simulink model "Storage_Cell"  (R2021b)
settings: Solver=VariableStepAuto  StartTime=0.0  StopTime=1  RelTol=1e-3
values from neighbouring files (symbols this model uses):
  dUdc = 0.1    [Storage_Cell_m.m]
  FFT_N = FFT_T / FFT_T_sample    (= 50)    [Storage_Cell_m.m]
  FFT_T_sample = 1/FFT_F_sample    (= 0.0002)    [Storage_Cell_m.m]
  Timesample = 1/(4*Fpwm)    (= 5e-05)    [Storage_Cell_m.m]
  Tpwm = 1/Fpwm    (= 0.0002)    [Storage_Cell_m.m]
  Udc = 450    [Storage_Cell_m.m]
  Us = 320    [Storage_Cell_m.m]
  Us_max = 380    [Storage_Cell_m.m]
libraries: spsSeriesRLCBranchLib x19, spsIGBTDiodeLib x10, spsVoltageMeasurementLib x10, spsSawtoothGeneratorLib x7, spsCurrentMeasurementLib x5, spsDCVoltageSourceLib x5, spspowerguiLib x1
settings Model: Creator=user  LastModifiedBy=mrsas

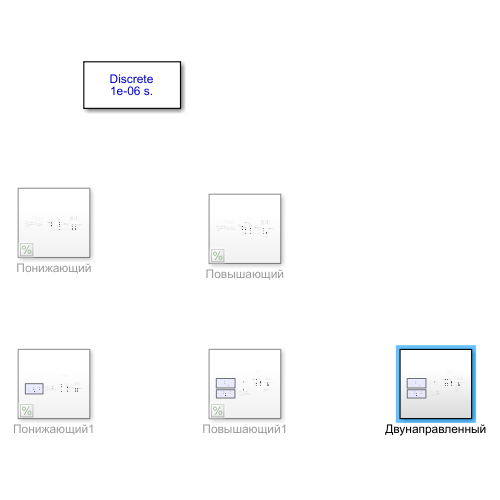
[thumbnail: Simulink's stored preview of the top-level diagram]
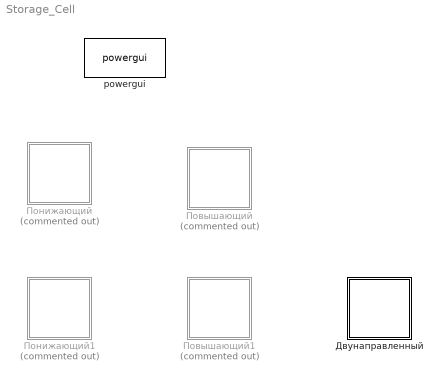
== system Storage_Cell ==
  powergui : spspowerguiLib/powergui  Priority=1  SimulationMode=Discrete  SampleTime=1e-6  frequency=60  Iterations=50  frequencyindice=0  Pbase=100e6  ErrMax=1e-4  UnitsV=kV  UnitsW=MW  buscounter=0  FunctionMessages=off  echomessages=off  EnableUseOfTLC=off  CurrentSourceSwitches=off  DisableSnubberDevices=off  DisableRonSwitches=off  DisableVfSwitches=off  DisplayEquations=off  AutomaticDiscreteSolvers=off  SolverType=Tustin/Backward Euler (TBE)  Interpol=off  ExternalGateDelay=off  methode=off  Ts=100  x0status=blocks  SPID=on  SwTol=0  HookPort=off  NonlinearTolerance=1e-4  nMaxIteration=100  ContinueOnMaxIteration=off  RestoreLinks=warning  ResistiveCurrentMeasurement=off  Frange=[0:2:500]  Ylog=off  Xlog=on  ShowGrid=off  save=off  variable=ZData  structure=0  ZoomFFT=off  StartTime=0.0  cycles=1  DisplayStyle=1  fundamental=60  FreqAxis=off  MaxFrequency=1000  frequencyindicesteady=1  RmsSteady=1  display=off
  Двунаправленный : Subsystem
  Повышающий : Subsystem  Commented=on
  Повышающий1 : Subsystem  Commented=on
  Понижающий : Subsystem  Commented=on
  Понижающий1 : Subsystem  Commented=on

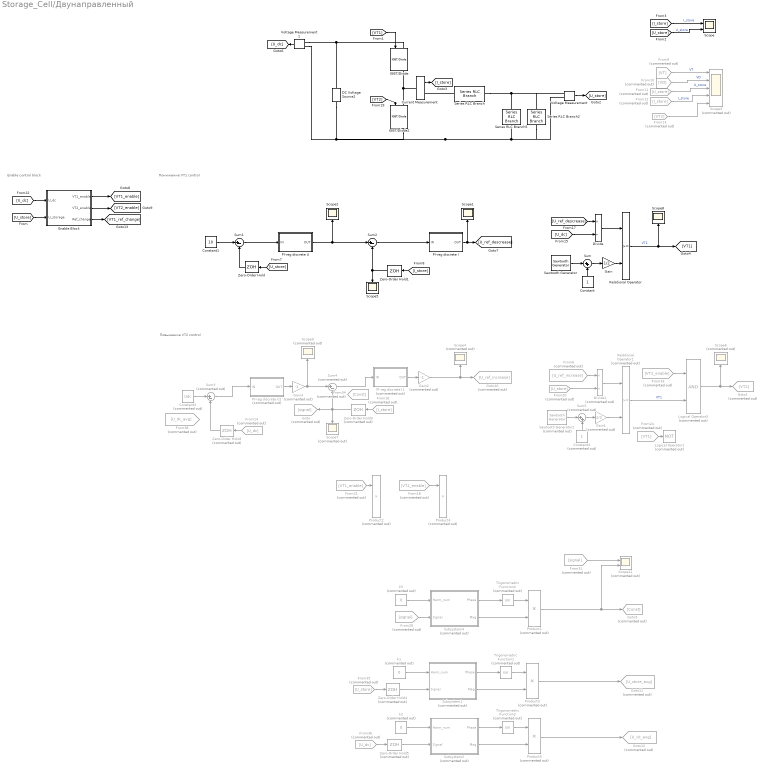
== system Storage_Cell/Двунаправленный ==
  note: Enable control block
  note: Повышение
      | VT2 control
  note: Понижение
      | VT1 control
  Constant : Constant
  Constant1 : Constant  Value=10
  Constant3 : Constant  Commented=on  Value=Udc
  Constant4 : Constant  Commented=on
  Current Measurement : spsCurrentMeasurementLib/Current Measurement  PhasorSimulation=off  OutputType=Complex  PSBequivalent=0
  DC Voltage Source2 : spsDCVoltageSourceLib/DC Voltage Source  Amplitude=20  Measurements=None
  Divide : Product  Inputs=*/
  Divide1 : Product  Commented=on  Inputs=*/
  Enable Block : Subsystem
  From10 : From  Commented=on  GotoTag=VD
  From11 : From  Commented=on  GotoTag=U_store
  From12 : From  Commented=on  GotoTag=I_store
  From13 : From  Commented=on  GotoTag=VT2
  From14 : From  Commented=on  GotoTag=U_dc
  From16 : From  Commented=on  GotoTag=I_store
  From18 : From  Commented=on  GotoTag=VT2_enable
  From20 : From  Commented=on  GotoTag=U_store
  From21 : From  Commented=on  GotoTag=VT1_enable
  From24 : From  Commented=on  GotoTag=VT1
  From28 : From  Commented=on  GotoTag=signal
  From31 : From  Commented=on  GotoTag=signal
  From33 : From  Commented=on  GotoTag=VT2_enable
  From34 : From  Commented=on  GotoTag=Const
  From35 : From  Commented=on  GotoTag=U_store
  From36 : From  Commented=on  GotoTag=U_dc
  From38 : From  Commented=on  GotoTag=U_dc_avg
  From6 : From  Commented=on  GotoTag=U_ref_increase
  From9 : From  Commented=on  GotoTag=VT
  Gain : Gain  Gain=1/2
  Gain1 : Gain  Commented=on  Gain=1/2
  Gain2 : Gain  Commented=on  Gain=-1
  Gain4 : Gain  Commented=on  Gain=-1
  Goto : Goto  Commented=on  GotoTag=signal
  Goto1 : Goto  Commented=on  GotoTag=VT2
  Goto10 : Goto  Commented=on  GotoTag=U_ref_increase
  Goto11 : Goto  Commented=on  GotoTag=U_store_avg
  Goto12 : Goto  Commented=on  GotoTag=U_dc_avg
  Goto5 : Goto  Commented=on  GotoTag=Const
  IGBT/Diode : spsIGBTDiodeLib/IGBT//Diode  Ron=1e-3  Rs=1e5  Cs=inf  Measurements=on
  IGBT/Diode2 : spsIGBTDiodeLib/IGBT//Diode  Ron=1e-3  Rs=1e5  Cs=inf  Measurements=on
  Logical Operator1 : Logic  Commented=on  Operator=NOT  AllPortsSameDT=off  OutDataTypeStr=boolean
  Logical Operator5 : Logic  Commented=on  AllPortsSameDT=off  OutDataTypeStr=boolean
  PI-reg discrete I : Subsystem  mask{First_condition=0, T=0.003, K=7.5, min=0, max=20, dt=Tpwm}
      mask prompts: T "Integral"; K "Proportional"; min "saturation_min"; max "saturation_max"; dt "timesample"
  PI-reg discrete I1 : Subsystem  Commented=on  mask{First_condition=370, T=0.001/0.1, K=3, min=-400, max=400, dt=Timesample}
      mask prompts: T "Integral"; K "Proportional"; min "saturation_min"; max "saturation_max"; dt "timesample"
  PI-reg discrete U : Subsystem  mask{First_condition=0, T=0.01, K=0.5, min=0, max=4, dt=Tpwm}
      mask prompts: T "Integral"; K "Proportional"; min "saturation_min"; max "saturation_max"; dt "timesample"
  PI-reg discrete U1 : Subsystem  Commented=on  mask{First_condition=0, T=0.1, K=0.1, min=-1000, max=1000, dt=Timesample}
      mask prompts: T "Integral"; K "Proportional"; min "saturation_min"; max "saturation_max"; dt "timesample"
  Product{1..5} (5 alike) : Product  Commented=on
  Relational Operator : RelationalOperator  OutDataTypeStr=boolean  RndMeth=Simplest
  Relational Operator1 : RelationalOperator  Commented=on  OutDataTypeStr=boolean  RndMeth=Simplest
  Sawtooth Generator : spsSawtoothGeneratorLib/Sawtooth Generator  Freq=Fpwm  Phase=0  Ts=0
  Sawtooth Generator1 : spsSawtoothGeneratorLib/Sawtooth Generator  Commented=on  Freq=Fpwm  Phase=0  Ts=0
  Scope : Scope  NumInputPorts=2
  Scope{1..2,5,8} (4 alike) : Scope
  Scope11 : Scope  Commented=on  NumInputPorts=2
  Scope3 : Scope  Commented=on  NumInputPorts=5
  Scope{4,6..7,9} (4 alike) : Scope  Commented=on
  Series RLC Branch : spsSeriesRLCBranchLib/Series RLC Branch  LConnTagsString=__new0  RConnTagsString=__new0  BranchType=RL  Resistance=0.1  Inductance=3e-3  SetiL0=on  InitialCurrent=0  Capacitance=1e-6  Setx0=off  InitialVoltage=0  Measurements=None
  Series RLC Branch2 : spsSeriesRLCBranchLib/Series RLC Branch  LConnTagsString=__new0  RConnTagsString=__new0  BranchType=R  Resistance=5  Inductance=1e-3  SetiL0=off  InitialCurrent=0  Capacitance=1000e-6  Setx0=on  InitialVoltage=0  Measurements=None
  Series RLC Branch5 : spsSeriesRLCBranchLib/Series RLC Branch  LConnTagsString=__new0  RConnTagsString=__new0  BranchType=C  Resistance=1  Inductance=1e-3  SetiL0=off  InitialCurrent=0  Capacitance=680e-6  Setx0=on  InitialVoltage=0  Measurements=None
  Subsystem1 : Subsystem  Commented=on
  Subsystem2 : Subsystem  Commented=on
  Subsystem4 : Subsystem  Commented=on
  Sum : Sum  Inputs=|++
  Sum1 : Sum  Inputs=|+-
  Sum2 : Sum  Inputs=|+-
  Sum3 : Sum  Commented=on  Inputs=|+-
  Sum4 : Sum  Commented=on  Inputs=|+-
  Sum5 : Sum  Commented=on  Inputs=|++
  Trigonometric Function1 : Trigonometry  Commented=on
  Trigonometric Function2 : Trigonometry  Commented=on
  Trigonometric Function4 : Trigonometry  Commented=on
  Voltage Measurement : spsVoltageMeasurementLib/Voltage Measurement  PhasorSimulation=off  OutputType=Complex  PSBequivalent=0
  Voltage Measurement1 : spsVoltageMeasurementLib/Voltage Measurement  PhasorSimulation=off  OutputType=Complex  PSBequivalent=0
  Zero-Order Hold : ZeroOrderHold  SampleTime=Timesample
  Zero-Order Hold1 : ZeroOrderHold  SampleTime=Timesample
  Zero-Order Hold{2..5} (4 alike) : ZeroOrderHold  Commented=on  SampleTime=Timesample
  k1 : Constant  Commented=on  Value=0
  k2 : Constant  Commented=on  Value=0
  k5 : Constant  Commented=on  Value=0
  wires:
  Gain2/1 -> Goto10/1, Scope4/1
  Gain4/1 -> Scope9/1, Sum4/1
  Divide1/1 -> Relational Operator1/1
  Sum3/1 -> PI-reg discrete U1/1(IN)
  Zero-Order Hold3/1 -> Sum4/2, Goto/1, Scope7/1
  PI-reg discrete U1/1(OUT) -> Gain4/1
  PI-reg discrete I1/1(OUT) -> Gain2/1
  Divide/1 -> Relational Operator/1
  Sum/1 -> Gain/1
  Current Measurement/1 -> [I_store]
  Gain/1 -> Relational Operator/2
  Sawtooth Generator/1 -> Sum/1
  Voltage Measurement1/1 -> [U_dc]
  Voltage Measurement/1 -> [U_store]
  Constant/1 -> Sum/2
  [U_ref_descrease] -> Divide/1
  Relational Operator/1 -> Scope8/1, [VT1]  "VT1"
  [VT1] -> IGBT/Diode/1
  PI-reg discrete I/1(OUT) -> [U_ref_descrease], Scope1/1
  [U_store] -> Zero-Order Hold/1
  Zero-Order Hold1/1 -> Scope5/1, Sum2/2
  [I_store] -> Zero-Order Hold1/1
  From9/1 -> Scope3/1  "VT"
  From10/1 -> Scope3/2  "VD"
  From11/1 -> Scope3/3  "U_store"
  From12/1 -> Scope3/4  "I_store"
  From13/1 -> Scope3/5
  Constant3/1 -> Sum3/1
  From14/1 -> Zero-Order Hold2/1
  Zero-Order Hold2/1 -> Sum3/2
  [U_dc] -> Divide/2
  From16/1 -> Zero-Order Hold3/1
  From20/1 -> Divide1/2
  From6/1 -> Divide1/1
  Constant4/1 -> Sum5/2
  Sawtooth Generator1/1 -> Sum5/1
  Gain1/1 -> Relational Operator1/2
  Sum5/1 -> Gain1/1
  [VT2] -> IGBT/Diode2/1
  [U_dc] -> Enable Block/1(U_dc)
  [U_store] -> Enable Block/2(U_storage)
  Enable Block/1(VT1_enable) -> [VT1_enable]
  Enable Block/2(VT2_enable) -> [VT2_enable]
  Enable Block/3(Ref_change) -> [VT1_ref_change]
  Sum1/1 -> PI-reg discrete U/1(IN)
  Constant1/1 -> Sum1/1
  Sum2/1 -> PI-reg discrete I/1(IN)
  Sum4/1 -> PI-reg discrete I1/1(IN)
  Relational Operator1/1 -> Logical Operator5/2  "VT1"
  From33/1 -> Logical Operator5/1
  Logical Operator5/1 -> Goto1/1, Scope6/1
  From18/1 -> Product4/1
  From21/1 -> Product2/1
  From24/1 -> Logical Operator1/1
  k5/1 -> Subsystem4/1(Harm_num)
  From28/1 -> Subsystem4/2(Signal)
  Product1/1 -> Scope11/2, Goto5/1
  Subsystem4/2(Mag) -> Product1/2
  Subsystem4/1(Phase) -> Trigonometric Function4/1
  Trigonometric Function4/1 -> Product1/1
  From31/1 -> Scope11/1
  From35/1 -> Zero-Order Hold4/1
  Trigonometric Function1/1 -> Product3/1
  Subsystem1/1(Phase) -> Trigonometric Function1/1
  Subsystem1/2(Mag) -> Product3/2
  Product3/1 -> Goto11/1
  Zero-Order Hold4/1 -> Subsystem1/2(Signal)
  k1/1 -> Subsystem1/1(Harm_num)
  k2/1 -> Subsystem2/1(Harm_num)
  Zero-Order Hold5/1 -> Subsystem2/2(Signal)
  Product5/1 -> Goto12/1
  Subsystem2/2(Mag) -> Product5/2
  Subsystem2/1(Phase) -> Trigonometric Function2/1
  Trigonometric Function2/1 -> Product5/1
  From36/1 -> Zero-Order Hold5/1
  Zero-Order Hold/1 -> Sum1/2
  PI-reg discrete U/1(OUT) -> Sum2/1, Scope2/1
  [I_store] -> Scope/1  "I_store"
  [U_store] -> Scope/2  "U_store"
  connections:
  Voltage Measurement1/LConn2 -- Series RLC Branch2/RConn1 -- Voltage Measurement/LConn2 -- Series RLC Branch5/RConn1 -- IGBT/Diode2/RConn1 -- DC Voltage Source2/LConn1
  Voltage Measurement1/LConn1 -- IGBT/Diode/LConn1 -- DC Voltage Source2/RConn1
  IGBT/Diode2/LConn1 -- Current Measurement/LConn1 -- IGBT/Diode/RConn1
  Series RLC Branch/LConn1 -- Current Measurement/RConn1
  Series RLC Branch2/LConn1 -- Voltage Measurement/LConn1 -- Series RLC Branch/RConn1 -- Series RLC Branch5/LConn1

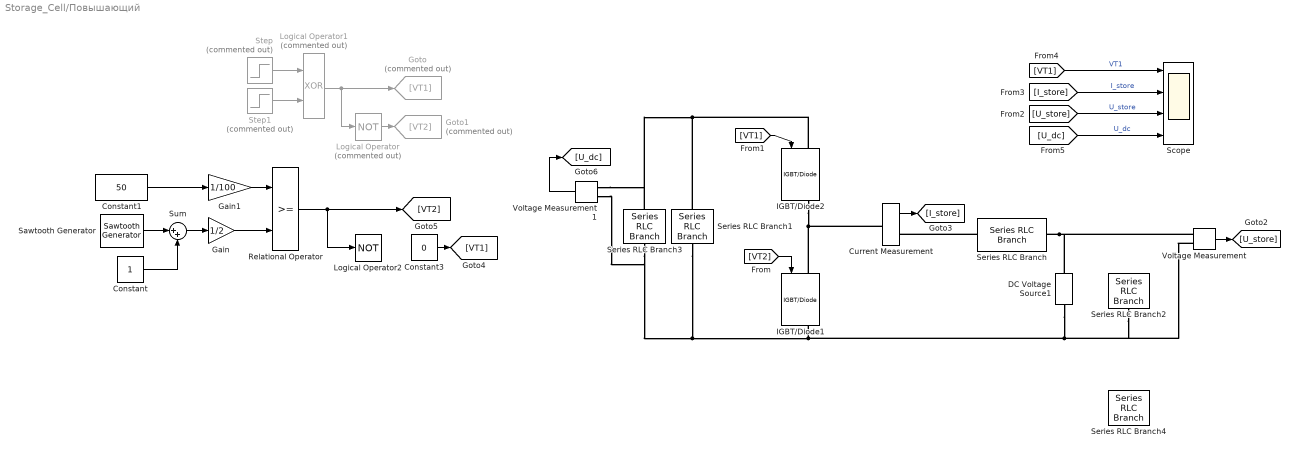
== system Storage_Cell/Повышающий ==
  Constant : Constant
  Constant1 : Constant  Value=50
  Constant3 : Constant  Value=0
  Current Measurement : spsCurrentMeasurementLib/Current Measurement  PhasorSimulation=off  OutputType=Complex  PSBequivalent=0
  DC Voltage Source1 : spsDCVoltageSourceLib/DC Voltage Source  Amplitude=100  Measurements=None
  Gain : Gain  Gain=1/2
  Gain1 : Gain  Gain=1/100
  Goto : Goto  Commented=on  GotoTag=VT1
  Goto1 : Goto  Commented=on  GotoTag=VT2
  IGBT/Diode1 : spsIGBTDiodeLib/IGBT//Diode  Ron=1e-3  Rs=1e5  Cs=inf  Measurements=on
  IGBT/Diode2 : spsIGBTDiodeLib/IGBT//Diode  Ron=1e-3  Rs=1e5  Cs=inf  Measurements=on
  Logical Operator : Logic  Commented=on  Operator=NOT  AllPortsSameDT=off  OutDataTypeStr=boolean
  Logical Operator1 : Logic  Commented=on  Operator=XOR  AllPortsSameDT=off  OutDataTypeStr=boolean
  Logical Operator2 : Logic  Operator=NOT  AllPortsSameDT=off  OutDataTypeStr=boolean
  Relational Operator : RelationalOperator  OutDataTypeStr=boolean  RndMeth=Simplest
  Sawtooth Generator : spsSawtoothGeneratorLib/Sawtooth Generator  Freq=10e3  Phase=0  Ts=0
  Scope : Scope  NumInputPorts=4
  Series RLC Branch : spsSeriesRLCBranchLib/Series RLC Branch  LConnTagsString=__new0  RConnTagsString=__new0  BranchType=RL  Resistance=0.1  Inductance=10e-3  SetiL0=on  InitialCurrent=0  Capacitance=1e-6  Setx0=off  InitialVoltage=0  Measurements=None
  Series RLC Branch1 : spsSeriesRLCBranchLib/Series RLC Branch  LConnTagsString=__new0  RConnTagsString=__new0  BranchType=R  Resistance=10  Inductance=1e-3  SetiL0=off  InitialCurrent=0  Capacitance=1000e-6  Setx0=on  InitialVoltage=0  Measurements=None
  Series RLC Branch2 : spsSeriesRLCBranchLib/Series RLC Branch  LConnTagsString=__new0  RConnTagsString=__new0  BranchType=R  Resistance=1  Inductance=1e-3  SetiL0=off  InitialCurrent=0  Capacitance=1000e-6  Setx0=on  InitialVoltage=0  Measurements=None
  Series RLC Branch3 : spsSeriesRLCBranchLib/Series RLC Branch  LConnTagsString=__new0  RConnTagsString=__new0  BranchType=C  Resistance=1  Inductance=1e-3  SetiL0=off  InitialCurrent=0  Capacitance=100e-6  Setx0=on  InitialVoltage=0  Measurements=None
  Series RLC Branch4 : spsSeriesRLCBranchLib/Series RLC Branch  LConnTagsString=__new0  RConnTagsString=__new0  BranchType=C  Resistance=1  Inductance=1e-3  SetiL0=off  InitialCurrent=0  Capacitance=100e-6  Setx0=on  InitialVoltage=0  Measurements=None
  Step : Step  Commented=on  Time=0.1  SampleTime=0
  Step1 : Step  Commented=on  Time=0.1+0.0002  SampleTime=0
  Sum : Sum  Inputs=|++
  Voltage Measurement : spsVoltageMeasurementLib/Voltage Measurement  PhasorSimulation=off  OutputType=Complex  PSBequivalent=0
  Voltage Measurement1 : spsVoltageMeasurementLib/Voltage Measurement  PhasorSimulation=off  OutputType=Complex  PSBequivalent=0
  wires:
  Step1/1 -> Logical Operator1/2
  Gain1/1 -> Relational Operator/1
  Sum/1 -> Gain/1
  Current Measurement/1 -> [I_store]
  Gain/1 -> Relational Operator/2
  [I_store] -> Scope/2  "I_store"
  Sawtooth Generator/1 -> Sum/1
  Voltage Measurement1/1 -> [U_dc]
  [U_store] -> Scope/3  "U_store"
  [VT1] -> Scope/1  "VT1"
  Voltage Measurement/1 -> [U_store]
  Logical Operator1/1 -> Goto/1, Logical Operator/1
  [VT2] -> IGBT/Diode1/1
  Step/1 -> Logical Operator1/1
  Logical Operator/1 -> Goto1/1
  Constant/1 -> Sum/2
  Constant1/1 -> Gain1/1
  Relational Operator/1 -> Logical Operator2/1, [VT2]
  [U_dc] -> Scope/4  "U_dc"
  [VT1] -> IGBT/Diode2/1
  Constant3/1 -> [VT1]
  connections:
  Series RLC Branch3/RConn1 -- Voltage Measurement1/LConn2 -- Series RLC Branch1/RConn1 -- IGBT/Diode1/RConn1 -- DC Voltage Source1/LConn1 -- Voltage Measurement/LConn2 -- Series RLC Branch2/RConn1
  Voltage Measurement1/LConn1 -- Series RLC Branch3/LConn1 -- IGBT/Diode2/LConn1 -- Series RLC Branch1/LConn1
  Current Measurement/LConn1 -- IGBT/Diode2/RConn1 -- IGBT/Diode1/LConn1
  Series RLC Branch/LConn1 -- Current Measurement/RConn1
  Series RLC Branch/RConn1 -- DC Voltage Source1/RConn1 -- Voltage Measurement/LConn1

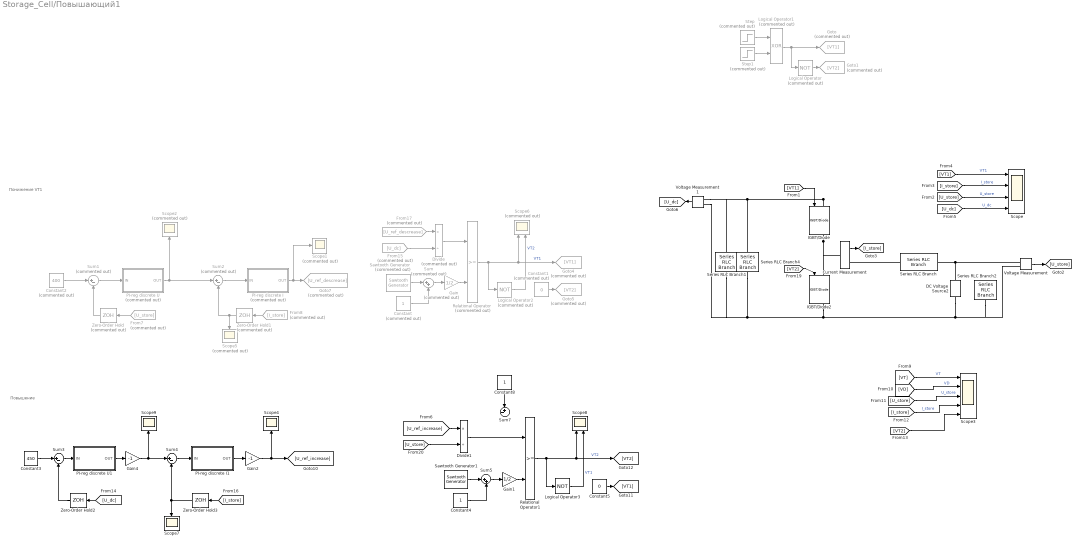
== system Storage_Cell/Повышающий1 ==
  note: Понижение
      | VT1
  note: Повышение
  Constant : Constant  Commented=on
  Constant1 : Constant  Commented=on  Value=0
  Constant2 : Constant  Commented=on  Value=400
  Constant3 : Constant  Value=450
  Constant4 : Constant
  Constant5 : Constant  Value=0
  Constant8 : Constant
  Current Measurement : spsCurrentMeasurementLib/Current Measurement  PhasorSimulation=off  OutputType=Complex  PSBequivalent=0
  DC Voltage Source2 : spsDCVoltageSourceLib/DC Voltage Source  Amplitude=400  Measurements=None
  Divide : Product  Commented=on  Inputs=*/
  Divide1 : Product  Inputs=*/
  From15 : From  Commented=on  GotoTag=U_dc
  From17 : From  Commented=on  GotoTag=U_ref_descrease
  From7 : From  Commented=on  GotoTag=U_store
  From8 : From  Commented=on  GotoTag=I_store
  Gain : Gain  Commented=on  Gain=1/2
  Gain1 : Gain  Gain=1/2
  Gain2 : Gain  Gain=-1
  Gain4 : Gain  Gain=-1
  Goto : Goto  Commented=on  GotoTag=VT1
  Goto1 : Goto  Commented=on  GotoTag=VT2
  Goto4 : Goto  Commented=on  GotoTag=VT1
  Goto5 : Goto  Commented=on  GotoTag=VT2
  Goto7 : Goto  Commented=on  GotoTag=U_ref_descrease
  IGBT/Diode : spsIGBTDiodeLib/IGBT//Diode  Ron=1e-3  Rs=1e5  Cs=inf  Measurements=on
  IGBT/Diode2 : spsIGBTDiodeLib/IGBT//Diode  Ron=1e-3  Rs=1e5  Cs=inf  Measurements=on
  Logical Operator : Logic  Commented=on  Operator=NOT  AllPortsSameDT=off  OutDataTypeStr=boolean
  Logical Operator1 : Logic  Commented=on  Operator=XOR  AllPortsSameDT=off  OutDataTypeStr=boolean
  Logical Operator2 : Logic  Commented=on  Operator=NOT  AllPortsSameDT=off  OutDataTypeStr=boolean
  Logical Operator3 : Logic  Operator=NOT  AllPortsSameDT=off  OutDataTypeStr=boolean
  PI-reg discrete I : Subsystem  Commented=on  mask{First_condition=0, T=0.001/0.1, K=10, min=0, max=450, dt=Timesample}
      mask prompts: T "Integral"; K "Proportional"; min "saturation_min"; max "saturation_max"; dt "timesample"
  PI-reg discrete I1 : Subsystem  mask{First_condition=400, T=0.001/0.1, K=3, min=-inf, max=400, dt=Timesample}
      mask prompts: T "Integral"; K "Proportional"; min "saturation_min"; max "saturation_max"; dt "timesample"
  PI-reg discrete U : Subsystem  Commented=on  mask{First_condition=0, T=0.1, K=0.1, min=-100, max=100, dt=Timesample}
      mask prompts: T "Integral"; K "Proportional"; min "saturation_min"; max "saturation_max"; dt "timesample"
  PI-reg discrete U1 : Subsystem  mask{First_condition=0, T=0.1, K=0.3, min=-50, max=100, dt=Timesample}
      mask prompts: T "Integral"; K "Proportional"; min "saturation_min"; max "saturation_max"; dt "timesample"
  Relational Operator : RelationalOperator  Commented=on  OutDataTypeStr=boolean  RndMeth=Simplest
  Relational Operator1 : RelationalOperator  OutDataTypeStr=boolean  RndMeth=Simplest
  Sawtooth Generator : spsSawtoothGeneratorLib/Sawtooth Generator  Commented=on  Freq=Fpwm  Phase=0  Ts=0
  Sawtooth Generator1 : spsSawtoothGeneratorLib/Sawtooth Generator  Freq=Fpwm  Phase=0  Ts=0
  Scope : Scope  NumInputPorts=4
  Scope1 : Scope  Commented=on
  Scope2 : Scope  Commented=on
  Scope3 : Scope  NumInputPorts=5
  Scope4 : Scope
  Scope5 : Scope  Commented=on
  Scope6 : Scope  Commented=on  NumInputPorts=2
  Scope7 : Scope
  Scope8 : Scope  NumInputPorts=2
  Scope9 : Scope
  Series RLC Branch : spsSeriesRLCBranchLib/Series RLC Branch  LConnTagsString=__new0  RConnTagsString=__new0  BranchType=RL  Resistance=0.1  Inductance=10e-3  SetiL0=on  InitialCurrent=0  Capacitance=1e-6  Setx0=off  InitialVoltage=0  Measurements=None
  Series RLC Branch1 : spsSeriesRLCBranchLib/Series RLC Branch  LConnTagsString=__new0  RConnTagsString=__new0  BranchType=R  Resistance=100  Inductance=1e-3  SetiL0=off  InitialCurrent=0  Capacitance=1000e-6  Setx0=on  InitialVoltage=0  Measurements=None
  Series RLC Branch2 : spsSeriesRLCBranchLib/Series RLC Branch  LConnTagsString=__new0  RConnTagsString=__new0  BranchType=R  Resistance=10000  Inductance=1e-3  SetiL0=off  InitialCurrent=0  Capacitance=1000e-6  Setx0=on  InitialVoltage=0  Measurements=None
  Series RLC Branch4 : spsSeriesRLCBranchLib/Series RLC Branch  LConnTagsString=__new0  RConnTagsString=__new0  BranchType=C  Resistance=1  Inductance=1e-3  SetiL0=off  InitialCurrent=0  Capacitance=100e-6  Setx0=on  InitialVoltage=300  Measurements=None
  Step : Step  Commented=on  Time=0.1  SampleTime=0
  Step1 : Step  Commented=on  Time=0.1+0.0002  SampleTime=0
  Sum : Sum  Commented=on  Inputs=|++
  Sum1 : Sum  Commented=on  Inputs=|+-
  Sum2 : Sum  Commented=on  Inputs=|+-
  Sum3 : Sum  Inputs=|+-
  Sum4 : Sum  Inputs=|+-
  Sum5 : Sum  Inputs=|++
  Sum7 : Sum  Inputs=+-|
  Voltage Measurement : spsVoltageMeasurementLib/Voltage Measurement  PhasorSimulation=off  OutputType=Complex  PSBequivalent=0
  Voltage Measurement1 : spsVoltageMeasurementLib/Voltage Measurement  PhasorSimulation=off  OutputType=Complex  PSBequivalent=0
  Zero-Order Hold : ZeroOrderHold  Commented=on  SampleTime=Timesample
  Zero-Order Hold1 : ZeroOrderHold  Commented=on  SampleTime=Timesample
  Zero-Order Hold2 : ZeroOrderHold  SampleTime=Timesample
  Zero-Order Hold3 : ZeroOrderHold  SampleTime=Timesample
  wires:
  [VT2] -> IGBT/Diode2/1
  Constant5/1 -> [VT1]
  Logical Operator3/1 -> Scope8/2  "VT1"
  Sum5/1 -> Gain1/1
  Gain1/1 -> Relational Operator1/2
  Sawtooth Generator1/1 -> Sum5/1
  Constant4/1 -> Sum5/2
  [U_ref_increase] -> Divide1/1
  Relational Operator1/1 -> Logical Operator3/1, Scope8/1, [VT2]  "VT2"
  [U_store] -> Divide1/2
  Sum4/1 -> PI-reg discrete I1/1(IN)
  [I_store] -> Zero-Order Hold3/1
  Constant1/1 -> Goto5/1
  From15/1 -> Divide/2
  Zero-Order Hold2/1 -> Sum3/2
  [U_dc] -> Zero-Order Hold2/1
  Constant3/1 -> Sum3/1
  [VT2] -> Scope3/5
  [I_store] -> Scope3/4  "I_store"
  [U_store] -> Scope3/3  "U_store"
  [VD] -> Scope3/2  "VD"
  [VT] -> Scope3/1  "VT"
  PI-reg discrete U/1(OUT) -> Scope2/1, Sum2/1
  From8/1 -> Zero-Order Hold1/1
  Zero-Order Hold1/1 -> Scope5/1, Sum2/2
  From7/1 -> Zero-Order Hold/1
  Zero-Order Hold/1 -> Sum1/2
  PI-reg discrete I/1(OUT) -> Goto7/1, Scope1/1
  Constant2/1 -> Sum1/1
  Sum2/1 -> PI-reg discrete I/1(IN)
  Sum1/1 -> PI-reg discrete U/1(IN)
  [VT1] -> IGBT/Diode/1
  [U_dc] -> Scope/4  "U_dc"
  Relational Operator/1 -> Scope6/1, Goto4/1, Logical Operator2/1  "VT1"
  From17/1 -> Divide/1
  Constant/1 -> Sum/2
  Logical Operator/1 -> Goto1/1
  Step/1 -> Logical Operator1/1
  Logical Operator1/1 -> Logical Operator/1, Goto/1
  Voltage Measurement/1 -> [U_store]
  [VT1] -> Scope/1  "VT1"
  [U_store] -> Scope/3  "U_store"
  Voltage Measurement1/1 -> [U_dc]
  Sawtooth Generator/1 -> Sum/1
  [I_store] -> Scope/2  "I_store"
  Gain/1 -> Relational Operator/2
  Current Measurement/1 -> [I_store]
  Sum/1 -> Gain/1
  Logical Operator2/1 -> Scope6/2  "VT2"
  Divide/1 -> Relational Operator/1
  Step1/1 -> Logical Operator1/2
  PI-reg discrete I1/1(OUT) -> Gain2/1
  PI-reg discrete U1/1(OUT) -> Gain4/1
  Zero-Order Hold3/1 -> Scope7/1, Sum4/2
  Sum3/1 -> PI-reg discrete U1/1(IN)
  Divide1/1 -> Relational Operator1/1
  Constant8/1 -> Sum7/1
  Gain4/1 -> Sum4/1, Scope9/1
  Gain2/1 -> [U_ref_increase], Scope4/1
  connections:
  Voltage Measurement/LConn1 -- DC Voltage Source2/RConn1 -- Series RLC Branch/RConn1
  Series RLC Branch/LConn1 -- Current Measurement/RConn1
  IGBT/Diode/RConn1 -- Current Measurement/LConn1 -- IGBT/Diode2/LConn1
  IGBT/Diode/LConn1 -- Series RLC Branch1/LConn1 -- Voltage Measurement1/LConn1 -- Series RLC Branch4/LConn1
  Voltage Measurement/LConn2 -- Series RLC Branch2/RConn1 -- IGBT/Diode2/RConn1 -- Voltage Measurement1/LConn2 -- Series RLC Branch1/RConn1 -- Series RLC Branch4/RConn1 -- DC Voltage Source2/LConn1

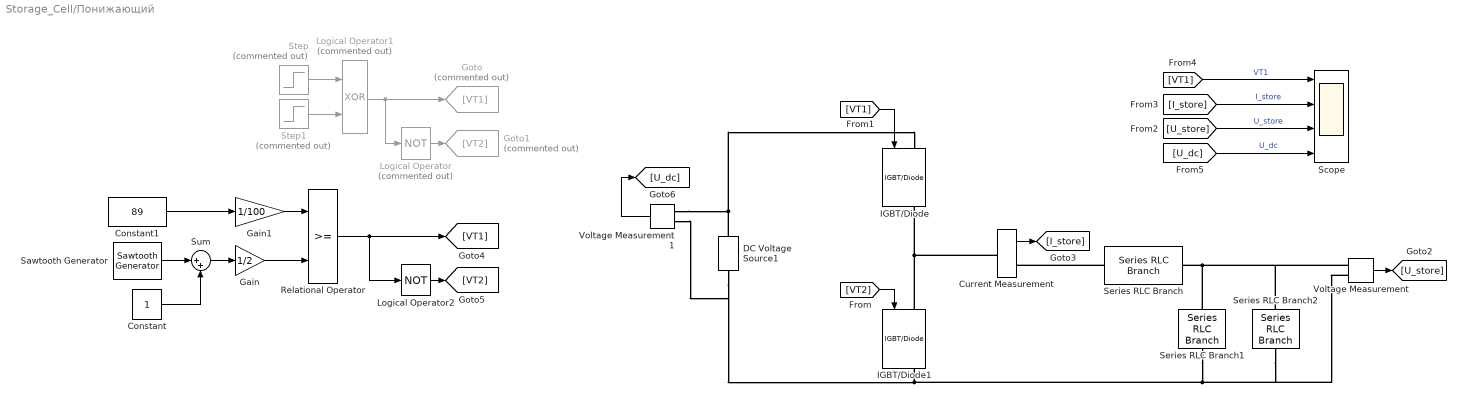
== system Storage_Cell/Понижающий ==
  Constant : Constant
  Constant1 : Constant  Value=89
  Current Measurement : spsCurrentMeasurementLib/Current Measurement  PhasorSimulation=off  OutputType=Complex  PSBequivalent=0
  DC Voltage Source1 : spsDCVoltageSourceLib/DC Voltage Source  Amplitude=450  Measurements=None
  Gain : Gain  Gain=1/2
  Gain1 : Gain  Gain=1/100
  Goto : Goto  Commented=on  GotoTag=VT1
  Goto1 : Goto  Commented=on  GotoTag=VT2
  IGBT/Diode : spsIGBTDiodeLib/IGBT//Diode  Ron=1e-3  Rs=1e5  Cs=inf  Measurements=on
  IGBT/Diode1 : spsIGBTDiodeLib/IGBT//Diode  Ron=1e-3  Rs=1e5  Cs=inf  Measurements=on
  Logical Operator : Logic  Commented=on  Operator=NOT  AllPortsSameDT=off  OutDataTypeStr=boolean
  Logical Operator1 : Logic  Commented=on  Operator=XOR  AllPortsSameDT=off  OutDataTypeStr=boolean
  Logical Operator2 : Logic  Operator=NOT  AllPortsSameDT=off  OutDataTypeStr=boolean
  Relational Operator : RelationalOperator  OutDataTypeStr=boolean  RndMeth=Simplest
  Sawtooth Generator : spsSawtoothGeneratorLib/Sawtooth Generator  Freq=10e3  Phase=0  Ts=0
  Scope : Scope  NumInputPorts=4
  Series RLC Branch : spsSeriesRLCBranchLib/Series RLC Branch  LConnTagsString=__new0  RConnTagsString=__new0  BranchType=RL  Resistance=0.1  Inductance=10e-3  SetiL0=on  InitialCurrent=0  Capacitance=1e-6  Setx0=off  InitialVoltage=0  Measurements=None
  Series RLC Branch1 : spsSeriesRLCBranchLib/Series RLC Branch  LConnTagsString=__new0  RConnTagsString=__new0  BranchType=C  Resistance=1  Inductance=1e-3  SetiL0=off  InitialCurrent=0  Capacitance=27e-6  Setx0=on  InitialVoltage=0  Measurements=None
  Series RLC Branch2 : spsSeriesRLCBranchLib/Series RLC Branch  LConnTagsString=__new0  RConnTagsString=__new0  BranchType=R  Resistance=10000  Inductance=1e-3  SetiL0=off  InitialCurrent=0  Capacitance=1000e-6  Setx0=on  InitialVoltage=0  Measurements=None
  Step : Step  Commented=on  Time=0.1  SampleTime=0
  Step1 : Step  Commented=on  Time=0.1+0.0002  SampleTime=0
  Sum : Sum  Inputs=|++
  Voltage Measurement : spsVoltageMeasurementLib/Voltage Measurement  PhasorSimulation=off  OutputType=Complex  PSBequivalent=0
  Voltage Measurement1 : spsVoltageMeasurementLib/Voltage Measurement  PhasorSimulation=off  OutputType=Complex  PSBequivalent=0
  wires:
  [VT1] -> IGBT/Diode/1
  [U_dc] -> Scope/4  "U_dc"
  Relational Operator/1 -> Logical Operator2/1, [VT1]
  Constant1/1 -> Gain1/1
  Constant/1 -> Sum/2
  Logical Operator/1 -> Goto1/1
  Step/1 -> Logical Operator1/1
  [VT2] -> IGBT/Diode1/1
  Logical Operator1/1 -> Logical Operator/1, Goto/1
  Voltage Measurement/1 -> [U_store]
  [VT1] -> Scope/1  "VT1"
  [U_store] -> Scope/3  "U_store"
  Voltage Measurement1/1 -> [U_dc]
  Sawtooth Generator/1 -> Sum/1
  [I_store] -> Scope/2  "I_store"
  Gain/1 -> Relational Operator/2
  Current Measurement/1 -> [I_store]
  Sum/1 -> Gain/1
  Logical Operator2/1 -> [VT2]
  Gain1/1 -> Relational Operator/1
  Step1/1 -> Logical Operator1/2
  connections:
  Series RLC Branch1/LConn1 -- Voltage Measurement/LConn1 -- Series RLC Branch2/LConn1 -- Series RLC Branch/RConn1
  Series RLC Branch/LConn1 -- Current Measurement/RConn1
  IGBT/Diode1/LConn1 -- IGBT/Diode/RConn1 -- Current Measurement/LConn1
  Voltage Measurement1/LConn1 -- DC Voltage Source1/RConn1 -- IGBT/Diode/LConn1
  Series RLC Branch1/RConn1 -- Series RLC Branch2/RConn1 -- Voltage Measurement/LConn2 -- DC Voltage Source1/LConn1 -- Voltage Measurement1/LConn2 -- IGBT/Diode1/RConn1

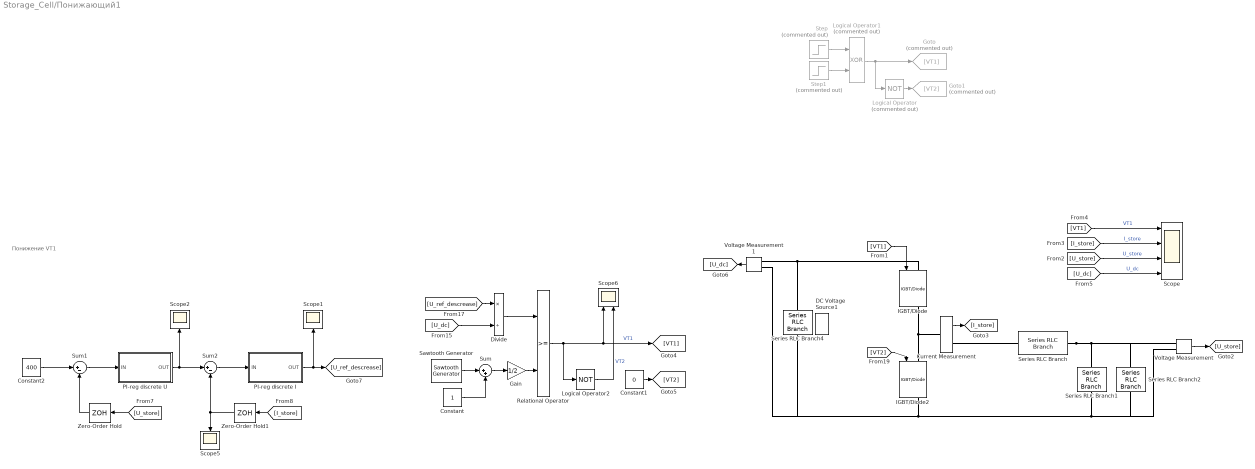
== system Storage_Cell/Понижающий1 ==
  note: Понижение
      | VT1
  Constant : Constant
  Constant1 : Constant  Value=0
  Constant2 : Constant  Value=400
  Current Measurement : spsCurrentMeasurementLib/Current Measurement  PhasorSimulation=off  OutputType=Complex  PSBequivalent=0
  DC Voltage Source1 : spsDCVoltageSourceLib/DC Voltage Source  Amplitude=450  Measurements=None
  Divide : Product  Inputs=*/
  Gain : Gain  Gain=1/2
  Goto : Goto  Commented=on  GotoTag=VT1
  Goto1 : Goto  Commented=on  GotoTag=VT2
  IGBT/Diode : spsIGBTDiodeLib/IGBT//Diode  Ron=1e-3  Rs=1e5  Cs=inf  Measurements=on
  IGBT/Diode2 : spsIGBTDiodeLib/IGBT//Diode  Ron=1e-3  Rs=1e5  Cs=inf  Measurements=on
  Logical Operator : Logic  Commented=on  Operator=NOT  AllPortsSameDT=off  OutDataTypeStr=boolean
  Logical Operator1 : Logic  Commented=on  Operator=XOR  AllPortsSameDT=off  OutDataTypeStr=boolean
  Logical Operator2 : Logic  Operator=NOT  AllPortsSameDT=off  OutDataTypeStr=boolean
  PI-reg discrete I : Subsystem  mask{First_condition=0, T=0.001/0.1, K=10, min=0, max=450, dt=Timesample}
      mask prompts: T "Integral"; K "Proportional"; min "saturation_min"; max "saturation_max"; dt "timesample"
  PI-reg discrete U : Subsystem  mask{First_condition=0, T=0.1, K=0.1, min=-100, max=100, dt=Timesample}
      mask prompts: T "Integral"; K "Proportional"; min "saturation_min"; max "saturation_max"; dt "timesample"
  Relational Operator : RelationalOperator  OutDataTypeStr=boolean  RndMeth=Simplest
  Sawtooth Generator : spsSawtoothGeneratorLib/Sawtooth Generator  Freq=Fpwm  Phase=0  Ts=0
  Scope : Scope  NumInputPorts=4
  Scope1 : Scope
  Scope2 : Scope
  Scope5 : Scope
  Scope6 : Scope  NumInputPorts=2
  Series RLC Branch : spsSeriesRLCBranchLib/Series RLC Branch  LConnTagsString=__new0  RConnTagsString=__new0  BranchType=RL  Resistance=0.1  Inductance=1e-3  SetiL0=on  InitialCurrent=0  Capacitance=1e-6  Setx0=off  InitialVoltage=0  Measurements=None
  Series RLC Branch1 : spsSeriesRLCBranchLib/Series RLC Branch  LConnTagsString=__new0  RConnTagsString=__new0  BranchType=C  Resistance=1  Inductance=1e-3  SetiL0=off  InitialCurrent=0  Capacitance=27e-6  Setx0=on  InitialVoltage=0  Measurements=None
  Series RLC Branch2 : spsSeriesRLCBranchLib/Series RLC Branch  LConnTagsString=__new0  RConnTagsString=__new0  BranchType=R  Resistance=10000  Inductance=1e-3  SetiL0=off  InitialCurrent=0  Capacitance=1000e-6  Setx0=on  InitialVoltage=0  Measurements=None
  Series RLC Branch4 : spsSeriesRLCBranchLib/Series RLC Branch  LConnTagsString=__new0  RConnTagsString=__new0  BranchType=C  Resistance=1  Inductance=1e-3  SetiL0=off  InitialCurrent=0  Capacitance=1000e-6  Setx0=on  InitialVoltage=450  Measurements=None
  Step : Step  Commented=on  Time=0.1  SampleTime=0
  Step1 : Step  Commented=on  Time=0.1+0.0002  SampleTime=0
  Sum : Sum  Inputs=|++
  Sum1 : Sum  Inputs=|+-
  Sum2 : Sum  Inputs=|+-
  Voltage Measurement : spsVoltageMeasurementLib/Voltage Measurement  PhasorSimulation=off  OutputType=Complex  PSBequivalent=0
  Voltage Measurement1 : spsVoltageMeasurementLib/Voltage Measurement  PhasorSimulation=off  OutputType=Complex  PSBequivalent=0
  Zero-Order Hold : ZeroOrderHold  SampleTime=Timesample
  Zero-Order Hold1 : ZeroOrderHold  SampleTime=Timesample
  wires:
  Step1/1 -> Logical Operator1/2
  Divide/1 -> Relational Operator/1
  Logical Operator2/1 -> Scope6/2  "VT2"
  Sum/1 -> Gain/1
  Current Measurement/1 -> [I_store]
  Gain/1 -> Relational Operator/2
  [I_store] -> Scope/2  "I_store"
  Sawtooth Generator/1 -> Sum/1
  Voltage Measurement1/1 -> [U_dc]
  [U_store] -> Scope/3  "U_store"
  [VT1] -> Scope/1  "VT1"
  Voltage Measurement/1 -> [U_store]
  Logical Operator1/1 -> Goto/1, Logical Operator/1
  Step/1 -> Logical Operator1/1
  Logical Operator/1 -> Goto1/1
  Constant/1 -> Sum/2
  [U_ref_descrease] -> Divide/1
  Relational Operator/1 -> Logical Operator2/1, [VT1], Scope6/1  "VT1"
  [U_dc] -> Scope/4  "U_dc"
  [VT1] -> IGBT/Diode/1
  Sum1/1 -> PI-reg discrete U/1(IN)
  Sum2/1 -> PI-reg discrete I/1(IN)
  Constant2/1 -> Sum1/1
  PI-reg discrete I/1(OUT) -> Scope1/1, [U_ref_descrease]
  Zero-Order Hold/1 -> Sum1/2
  [U_store] -> Zero-Order Hold/1
  Zero-Order Hold1/1 -> Sum2/2, Scope5/1
  [I_store] -> Zero-Order Hold1/1
  PI-reg discrete U/1(OUT) -> Sum2/1, Scope2/1
  [U_dc] -> Divide/2
  Constant1/1 -> [VT2]
  [VT2] -> IGBT/Diode2/1
  connections:
  Series RLC Branch4/RConn1 -- Voltage Measurement1/LConn2 -- Series RLC Branch2/RConn1 -- Voltage Measurement/LConn2 -- Series RLC Branch1/RConn1 -- IGBT/Diode2/RConn1
  Voltage Measurement1/LConn1 -- IGBT/Diode/LConn1 -- Series RLC Branch4/LConn1
  Current Measurement/LConn1 -- IGBT/Diode2/LConn1 -- IGBT/Diode/RConn1
  Series RLC Branch/LConn1 -- Current Measurement/RConn1
  Series RLC Branch/RConn1 -- Voltage Measurement/LConn1 -- Series RLC Branch2/LConn1 -- Series RLC Branch1/LConn1

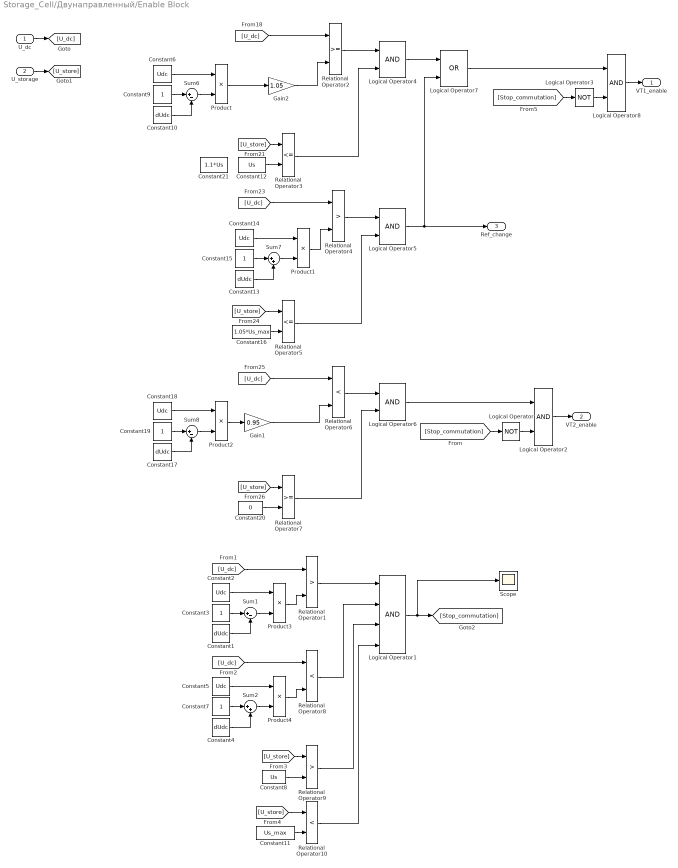
== system Storage_Cell/Двунаправленный/Enable Block ==
  U_dc : Inport
  U_storage : Inport  Port=2
  Constant{1,4,10,13,17} (5 alike) : Constant  Value=dUdc
  Constant11 : Constant  Value=Us_max
  Constant12 : Constant  Value=Us
  Constant{2,5..6,14,18} (5 alike) : Constant  Value=Udc
  Constant{3,7,9,15,19} (5 alike) : Constant
  Constant16 : Constant  Value=1.05*Us_max
  Constant20 : Constant  Value=0
  Constant21 : Constant  Value=1.1*Us
  Constant8 : Constant  Value=Us
  Gain1 : Gain  Gain=0.95
  Gain2 : Gain  Gain=1.05
  Logical Operator : Logic  Operator=NOT  AllPortsSameDT=off  OutDataTypeStr=boolean
  Logical Operator1 : Logic  Inputs=4  AllPortsSameDT=off  OutDataTypeStr=boolean
  Logical Operator{2,4..6,8} (5 alike) : Logic  AllPortsSameDT=off  OutDataTypeStr=boolean
  Logical Operator3 : Logic  Operator=NOT  AllPortsSameDT=off  OutDataTypeStr=boolean
  Logical Operator7 : Logic  Operator=OR  AllPortsSameDT=off  OutDataTypeStr=boolean
  Product{,1..4} (5 alike) : Product
  Relational Operator1 : RelationalOperator  Operator=>  OutDataTypeStr=boolean  RndMeth=Simplest
  Relational Operator10 : RelationalOperator  Operator=<  OutDataTypeStr=boolean  RndMeth=Simplest
  Relational Operator2 : RelationalOperator  OutDataTypeStr=boolean  RndMeth=Simplest
  Relational Operator3 : RelationalOperator  Operator=<=  OutDataTypeStr=boolean  RndMeth=Simplest
  Relational Operator4 : RelationalOperator  Operator=>  OutDataTypeStr=boolean  RndMeth=Simplest
  Relational Operator5 : RelationalOperator  Operator=<=  OutDataTypeStr=boolean  RndMeth=Simplest
  Relational Operator6 : RelationalOperator  Operator=<  OutDataTypeStr=boolean  RndMeth=Simplest
  Relational Operator7 : RelationalOperator  OutDataTypeStr=boolean  RndMeth=Simplest
  Relational Operator8 : RelationalOperator  Operator=<  OutDataTypeStr=boolean  RndMeth=Simplest
  Relational Operator9 : RelationalOperator  Operator=>  OutDataTypeStr=boolean  RndMeth=Simplest
  Scope : Scope
  Sum1 : Sum  Inputs=|+-
  Sum2 : Sum  Inputs=|++
  Sum6 : Sum  Inputs=|+-
  Sum7 : Sum  Inputs=|++
  Sum8 : Sum  Inputs=|+-
  VT1_enable : Outport
  VT2_enable : Outport  Port=2
  Ref_change : Outport  Port=3
  wires:
  [U_dc] -> Relational Operator6/1
  [U_store] -> Relational Operator3/1
  Constant15/1 -> Sum7/1
  Logical Operator5/1 -> Ref_change/1, Logical Operator7/2
  Logical Operator4/1 -> Logical Operator7/1
  Constant6/1 -> Product/1
  Constant18/1 -> Product2/1
  Constant9/1 -> Sum6/1
  Constant14/1 -> Product1/1
  Constant12/1 -> Relational Operator3/2
  Constant20/1 -> Relational Operator7/2
  Relational Operator3/1 -> Logical Operator4/2
  [U_dc] -> Relational Operator4/1
  Sum7/1 -> Product1/2
  Constant10/1 -> Sum6/2
  Constant13/1 -> Sum7/2
  Constant19/1 -> Sum8/1
  Constant17/1 -> Sum8/2
  [U_store] -> Relational Operator5/1
  Logical Operator6/1 -> Logical Operator2/1
  Relational Operator7/1 -> Logical Operator6/2
  Relational Operator6/1 -> Logical Operator6/1
  [U_dc] -> Relational Operator2/1
  [U_store] -> Relational Operator7/1
  Gain1/1 -> Relational Operator6/2
  Sum6/1 -> Product/2
  Sum8/1 -> Product2/2
  Relational Operator5/1 -> Logical Operator5/2
  Product/1 -> Gain2/1
  Relational Operator2/1 -> Logical Operator4/1
  Relational Operator4/1 -> Logical Operator5/1
  Constant16/1 -> Relational Operator5/2
  U_dc/1 -> [U_dc]
  U_storage/1 -> [U_store]
  Product1/1 -> Relational Operator4/2
  Product2/1 -> Gain1/1
  Gain2/1 -> Relational Operator2/2
  Product3/1 -> Relational Operator1/2
  Sum1/1 -> Product3/2
  [U_dc] -> Relational Operator1/1
  Constant1/1 -> Sum1/2
  Constant3/1 -> Sum1/1
  Constant2/1 -> Product3/1
  Constant5/1 -> Product4/1
  Constant7/1 -> Sum2/1
  Constant4/1 -> Sum2/2
  [U_dc] -> Relational Operator8/1
  Sum2/1 -> Product4/2
  Product4/1 -> Relational Operator8/2
  [U_store] -> Relational Operator9/1
  Constant8/1 -> Relational Operator9/2
  Constant11/1 -> Relational Operator10/2
  [U_store] -> Relational Operator10/1
  Relational Operator1/1 -> Logical Operator1/1
  Relational Operator8/1 -> Logical Operator1/2
  Relational Operator9/1 -> Logical Operator1/3
  Relational Operator10/1 -> Logical Operator1/4
  Logical Operator1/1 -> Scope/1, [Stop_commutation]
  [Stop_commutation] -> Logical Operator/1
  Logical Operator2/1 -> VT2_enable/1
  Logical Operator/1 -> Logical Operator2/2
  Logical Operator3/1 -> Logical Operator8/2
  [Stop_commutation] -> Logical Operator3/1
  Logical Operator7/1 -> Logical Operator8/1
  Logical Operator8/1 -> VT1_enable/1

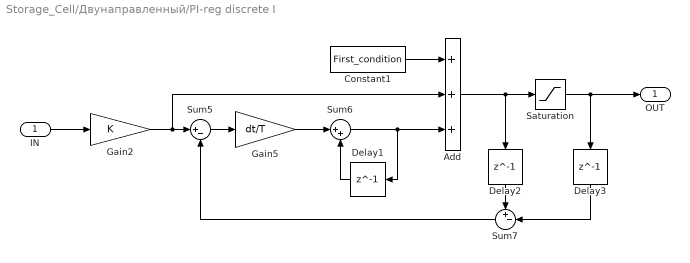
== system Storage_Cell/Двунаправленный/PI-reg discrete I ==
  IN : Inport
  Add : Sum  Inputs=+++
  Constant1 : Constant  Value=First_condition
  Delay1 : Delay  DelayLength=1  InitialCondition=0  SampleTime=dt
  Delay2 : Delay  DelayLength=1  InitialCondition=0  SampleTime=dt
  Delay3 : Delay  DelayLength=1  InitialCondition=0  SampleTime=dt
  Gain2 : Gain  Gain=K
  Gain5 : Gain  Gain=dt/T
  Saturation : Saturate  UpperLimit=max  LowerLimit=min
  Sum5 : Sum  Inputs=|+-
  Sum6 : Sum  Inputs=|++
  Sum7 : Sum  Inputs=+-|
  OUT : Outport
  wires:
  Delay2/1 -> Sum7/1
  Sum7/1 -> Sum5/2
  Delay1/1 -> Sum6/2
  Sum5/1 -> Gain5/1
  Delay3/1 -> Sum7/2
  Gain5/1 -> Sum6/1
  Gain2/1 -> Add/2, Sum5/1
  Saturation/1 -> Delay3/1, OUT/1
  Sum6/1 -> Add/3, Delay1/1
  Add/1 -> Saturation/1, Delay2/1
  IN/1 -> Gain2/1
  Constant1/1 -> Add/1

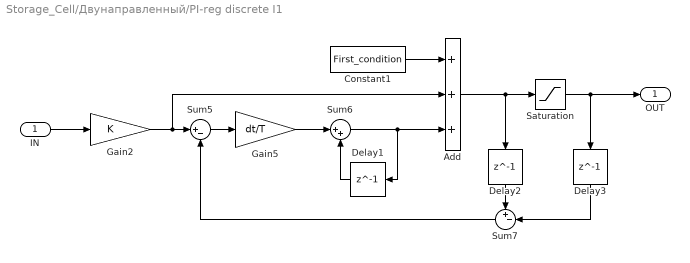
== system Storage_Cell/Двунаправленный/PI-reg discrete I1 ==
  IN : Inport
  Add : Sum  Inputs=+++
  Constant1 : Constant  Value=First_condition
  Delay1 : Delay  DelayLength=1  InitialCondition=0  SampleTime=dt
  Delay2 : Delay  DelayLength=1  InitialCondition=0  SampleTime=dt
  Delay3 : Delay  DelayLength=1  InitialCondition=0  SampleTime=dt
  Gain2 : Gain  Gain=K
  Gain5 : Gain  Gain=dt/T
  Saturation : Saturate  UpperLimit=max  LowerLimit=min
  Sum5 : Sum  Inputs=|+-
  Sum6 : Sum  Inputs=|++
  Sum7 : Sum  Inputs=+-|
  OUT : Outport
  wires:
  Constant1/1 -> Add/1
  IN/1 -> Gain2/1
  Add/1 -> Delay2/1, Saturation/1
  Sum6/1 -> Delay1/1, Add/3
  Saturation/1 -> OUT/1, Delay3/1
  Gain2/1 -> Sum5/1, Add/2
  Gain5/1 -> Sum6/1
  Delay3/1 -> Sum7/2
  Sum5/1 -> Gain5/1
  Delay1/1 -> Sum6/2
  Sum7/1 -> Sum5/2
  Delay2/1 -> Sum7/1

== system Storage_Cell/Двунаправленный/PI-reg discrete U ==
  IN : Inport
  Add : Sum  Inputs=+++
  Constant1 : Constant  Value=First_condition
  Delay1 : Delay  DelayLength=1  InitialCondition=0  SampleTime=dt
  Delay2 : Delay  DelayLength=1  InitialCondition=0  SampleTime=dt
  Delay3 : Delay  DelayLength=1  InitialCondition=0  SampleTime=dt
  Gain2 : Gain  Gain=K
  Gain5 : Gain  Gain=dt/T
  Saturation : Saturate  UpperLimit=max  LowerLimit=min
  Sum5 : Sum  Inputs=|+-
  Sum6 : Sum  Inputs=|++
  Sum7 : Sum  Inputs=+-|
  OUT : Outport
  wires:
  Constant1/1 -> Add/1
  IN/1 -> Gain2/1
  Add/1 -> Delay2/1, Saturation/1
  Sum6/1 -> Delay1/1, Add/3
  Saturation/1 -> OUT/1, Delay3/1
  Gain2/1 -> Sum5/1, Add/2
  Gain5/1 -> Sum6/1
  Delay3/1 -> Sum7/2
  Sum5/1 -> Gain5/1
  Delay1/1 -> Sum6/2
  Sum7/1 -> Sum5/2
  Delay2/1 -> Sum7/1

== system Storage_Cell/Двунаправленный/PI-reg discrete U1 ==
  IN : Inport
  Add : Sum  Inputs=+++
  Constant1 : Constant  Value=First_condition
  Delay1 : Delay  DelayLength=1  InitialCondition=0  SampleTime=dt
  Delay2 : Delay  DelayLength=1  InitialCondition=0  SampleTime=dt
  Delay3 : Delay  DelayLength=1  InitialCondition=0  SampleTime=dt
  Gain2 : Gain  Gain=K
  Gain5 : Gain  Gain=dt/T
  Saturation : Saturate  UpperLimit=max  LowerLimit=min
  Sum5 : Sum  Inputs=|+-
  Sum6 : Sum  Inputs=|++
  Sum7 : Sum  Inputs=+-|
  OUT : Outport
  wires:
  Delay2/1 -> Sum7/1
  Sum7/1 -> Sum5/2
  Delay1/1 -> Sum6/2
  Sum5/1 -> Gain5/1
  Delay3/1 -> Sum7/2
  Gain5/1 -> Sum6/1
  Gain2/1 -> Add/2, Sum5/1
  Saturation/1 -> Delay3/1, OUT/1
  Sum6/1 -> Add/3, Delay1/1
  Add/1 -> Saturation/1, Delay2/1
  IN/1 -> Gain2/1
  Constant1/1 -> Add/1

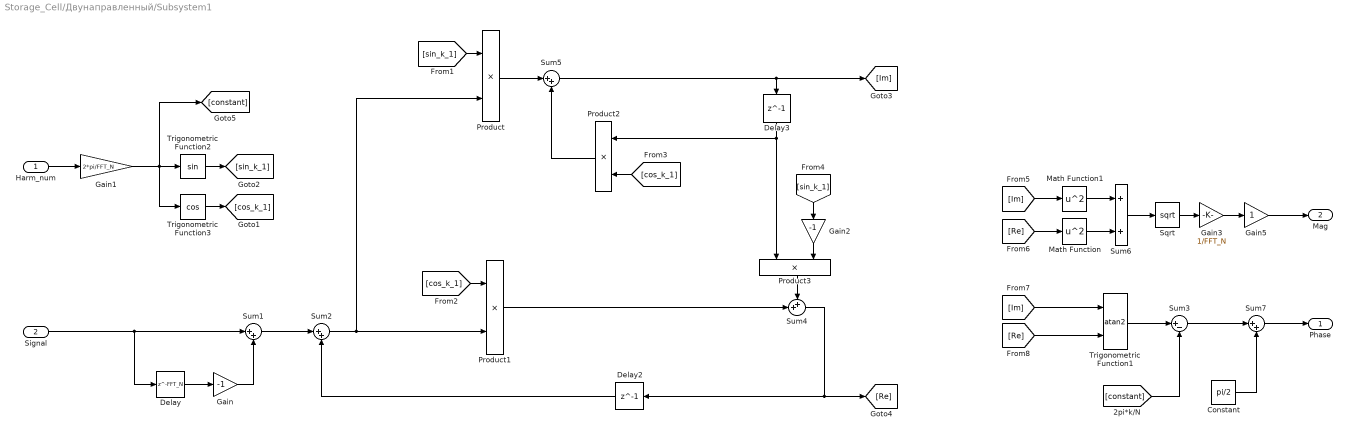
== system Storage_Cell/Двунаправленный/Subsystem1 ==
  Harm_num : Inport
  Signal : Inport  Port=2
  Constant : Constant  Value=pi/2
  Delay : Delay  DelayLength=FFT_N  SampleTime=FFT_T_sample
  Delay2 : Delay  DelayLength=1  SampleTime=FFT_T_sample
  Delay3 : Delay  DelayLength=1  SampleTime=FFT_T_sample
  Gain : Gain  Gain=-1
  Gain1 : Gain  Gain=2*pi/FFT_N
  Gain2 : Gain  Gain=-1
  Gain3 : Gain  Gain=1/FFT_N
  Gain5 : Gain
  Math Function : Math  Operator=square  SaturateOnIntegerOverflow=on
  Math Function1 : Math  Operator=square  SaturateOnIntegerOverflow=on
  Product{,1..3} (4 alike) : Product
  Sqrt : Sqrt  SaturateOnIntegerOverflow=on
  Sum{1..2,5,7} (4 alike) : Sum  Inputs=|++
  Sum3 : Sum  Inputs=|+-
  Sum4 : Sum  Inputs=++|
  Sum6 : Sum
  Trigonometric Function1 : Trigonometry  Operator=atan2
  Trigonometric Function2 : Trigonometry
  Trigonometric Function3 : Trigonometry  Operator=cos
  Phase : Outport
  Mag : Outport  Port=2
  wires:
  [sin_k_1] -> Gain2/1
  Sum5/1 -> [Im], Delay3/1
  Sum3/1 -> Sum7/1
  Product2/1 -> Sum5/2
  Math Function1/1 -> Sum6/1
  Product/1 -> Sum5/1
  Sum2/1 -> Product/2, Product1/2
  [Re] -> Math Function/1
  Delay3/1 -> Product2/1, Product3/1
  Trigonometric Function3/1 -> [cos_k_1]
  Sum6/1 -> Sqrt/1
  Gain/1 -> Sum1/2
  Delay/1 -> Gain/1
  Gain5/1 -> Mag/1
  Signal/1 -> Sum1/1, Delay/1
  Gain1/1 -> [constant], Trigonometric Function3/1, Trigonometric Function2/1
  Product3/1 -> Sum4/1
  Gain3/1 -> Gain5/1
  Sqrt/1 -> Gain3/1
  [Im] -> Math Function1/1
  Product1/1 -> Sum4/2
  [cos_k_1] -> Product2/2
  [sin_k_1] -> Product/1
  Sum4/1 -> [Re], Delay2/1
  Math Function/1 -> Sum6/2
  Delay2/1 -> Sum2/2
  [cos_k_1] -> Product1/1
  Gain2/1 -> Product3/2
  Trigonometric Function2/1 -> [sin_k_1]
  [Re] -> Trigonometric Function1/2
  Sum1/1 -> Sum2/1
  Harm_num/1 -> Gain1/1
  Trigonometric Function1/1 -> Sum3/1
  [Im] -> Trigonometric Function1/1
  Sum7/1 -> Phase/1
  Constant/1 -> Sum7/2
  [constant] -> Sum3/2

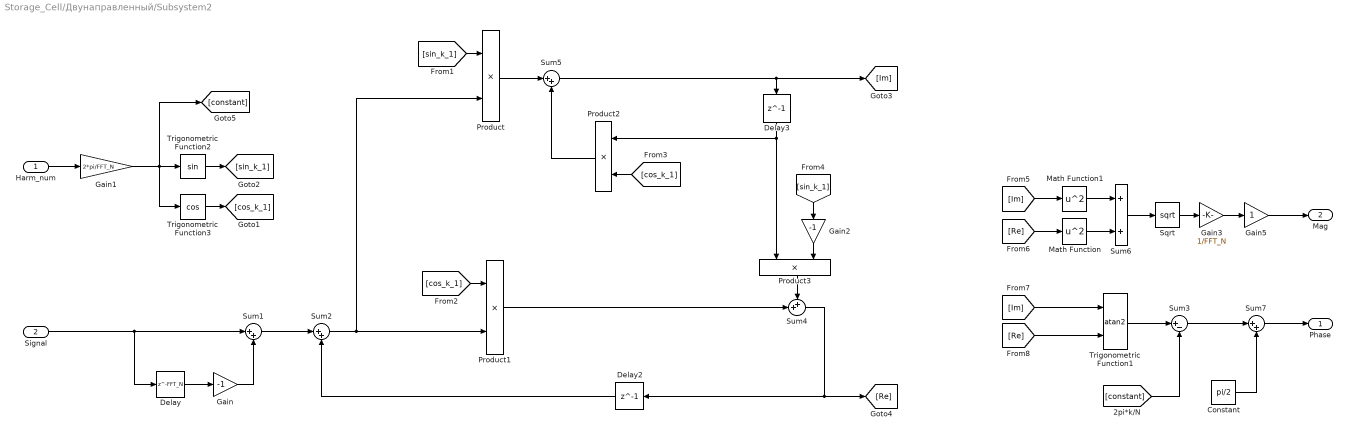
== system Storage_Cell/Двунаправленный/Subsystem2 ==
  Harm_num : Inport
  Signal : Inport  Port=2
  Constant : Constant  Value=pi/2
  Delay : Delay  DelayLength=FFT_N  SampleTime=FFT_T_sample
  Delay2 : Delay  DelayLength=1  SampleTime=FFT_T_sample
  Delay3 : Delay  DelayLength=1  SampleTime=FFT_T_sample
  Gain : Gain  Gain=-1
  Gain1 : Gain  Gain=2*pi/FFT_N
  Gain2 : Gain  Gain=-1
  Gain3 : Gain  Gain=1/FFT_N
  Gain5 : Gain
  Math Function : Math  Operator=square  SaturateOnIntegerOverflow=on
  Math Function1 : Math  Operator=square  SaturateOnIntegerOverflow=on
  Product{,1..3} (4 alike) : Product
  Sqrt : Sqrt  SaturateOnIntegerOverflow=on
  Sum{1..2,5,7} (4 alike) : Sum  Inputs=|++
  Sum3 : Sum  Inputs=|+-
  Sum4 : Sum  Inputs=++|
  Sum6 : Sum
  Trigonometric Function1 : Trigonometry  Operator=atan2
  Trigonometric Function2 : Trigonometry
  Trigonometric Function3 : Trigonometry  Operator=cos
  Phase : Outport
  Mag : Outport  Port=2
  wires:
  [constant] -> Sum3/2
  Constant/1 -> Sum7/2
  Sum7/1 -> Phase/1
  [Im] -> Trigonometric Function1/1
  Trigonometric Function1/1 -> Sum3/1
  Harm_num/1 -> Gain1/1
  Sum1/1 -> Sum2/1
  [Re] -> Trigonometric Function1/2
  Trigonometric Function2/1 -> [sin_k_1]
  Gain2/1 -> Product3/2
  [cos_k_1] -> Product1/1
  Delay2/1 -> Sum2/2
  Math Function/1 -> Sum6/2
  Sum4/1 -> Delay2/1, [Re]
  [sin_k_1] -> Product/1
  [cos_k_1] -> Product2/2
  Product1/1 -> Sum4/2
  [Im] -> Math Function1/1
  Sqrt/1 -> Gain3/1
  Gain3/1 -> Gain5/1
  Product3/1 -> Sum4/1
  Gain1/1 -> Trigonometric Function2/1, Trigonometric Function3/1, [constant]
  Signal/1 -> Delay/1, Sum1/1
  Gain5/1 -> Mag/1
  Delay/1 -> Gain/1
  Gain/1 -> Sum1/2
  Sum6/1 -> Sqrt/1
  Trigonometric Function3/1 -> [cos_k_1]
  Delay3/1 -> Product3/1, Product2/1
  [Re] -> Math Function/1
  Sum2/1 -> Product1/2, Product/2
  Product/1 -> Sum5/1
  Math Function1/1 -> Sum6/1
  Product2/1 -> Sum5/2
  Sum3/1 -> Sum7/1
  Sum5/1 -> Delay3/1, [Im]
  [sin_k_1] -> Gain2/1

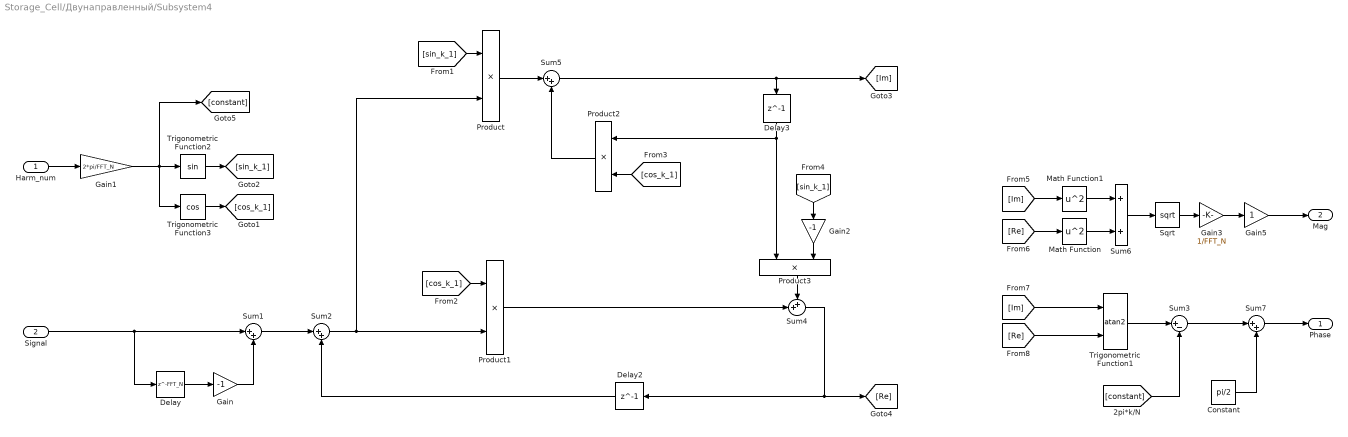
== system Storage_Cell/Двунаправленный/Subsystem4 ==
  Harm_num : Inport
  Signal : Inport  Port=2
  Constant : Constant  Value=pi/2
  Delay : Delay  DelayLength=FFT_N  SampleTime=FFT_T_sample
  Delay2 : Delay  DelayLength=1  SampleTime=FFT_T_sample
  Delay3 : Delay  DelayLength=1  SampleTime=FFT_T_sample
  Gain : Gain  Gain=-1
  Gain1 : Gain  Gain=2*pi/FFT_N
  Gain2 : Gain  Gain=-1
  Gain3 : Gain  Gain=1/FFT_N
  Gain5 : Gain
  Math Function : Math  Operator=square  SaturateOnIntegerOverflow=on
  Math Function1 : Math  Operator=square  SaturateOnIntegerOverflow=on
  Product{,1..3} (4 alike) : Product
  Sqrt : Sqrt  SaturateOnIntegerOverflow=on
  Sum{1..2,5,7} (4 alike) : Sum  Inputs=|++
  Sum3 : Sum  Inputs=|+-
  Sum4 : Sum  Inputs=++|
  Sum6 : Sum
  Trigonometric Function1 : Trigonometry  Operator=atan2
  Trigonometric Function2 : Trigonometry
  Trigonometric Function3 : Trigonometry  Operator=cos
  Phase : Outport
  Mag : Outport  Port=2
  wires:
  [constant] -> Sum3/2
  Constant/1 -> Sum7/2
  Sum7/1 -> Phase/1
  [Im] -> Trigonometric Function1/1
  Trigonometric Function1/1 -> Sum3/1
  Harm_num/1 -> Gain1/1
  Sum1/1 -> Sum2/1
  [Re] -> Trigonometric Function1/2
  Trigonometric Function2/1 -> [sin_k_1]
  Gain2/1 -> Product3/2
  [cos_k_1] -> Product1/1
  Delay2/1 -> Sum2/2
  Math Function/1 -> Sum6/2
  Sum4/1 -> Delay2/1, [Re]
  [sin_k_1] -> Product/1
  [cos_k_1] -> Product2/2
  Product1/1 -> Sum4/2
  [Im] -> Math Function1/1
  Sqrt/1 -> Gain3/1
  Gain3/1 -> Gain5/1
  Product3/1 -> Sum4/1
  Gain1/1 -> Trigonometric Function2/1, Trigonometric Function3/1, [constant]
  Signal/1 -> Delay/1, Sum1/1
  Gain5/1 -> Mag/1
  Delay/1 -> Gain/1
  Gain/1 -> Sum1/2
  Sum6/1 -> Sqrt/1
  Trigonometric Function3/1 -> [cos_k_1]
  Delay3/1 -> Product3/1, Product2/1
  [Re] -> Math Function/1
  Sum2/1 -> Product1/2, Product/2
  Product/1 -> Sum5/1
  Math Function1/1 -> Sum6/1
  Product2/1 -> Sum5/2
  Sum3/1 -> Sum7/1
  Sum5/1 -> Delay3/1, [Im]
  [sin_k_1] -> Gain2/1

== system Storage_Cell/Повышающий1/PI-reg discrete I ==
  IN : Inport
  Add : Sum  Inputs=+++
  Constant1 : Constant  Value=First_condition
  Delay1 : Delay  DelayLength=1  InitialCondition=0  SampleTime=dt
  Delay2 : Delay  DelayLength=1  InitialCondition=0  SampleTime=dt
  Delay3 : Delay  DelayLength=1  InitialCondition=0  SampleTime=dt
  Gain2 : Gain  Gain=K
  Gain5 : Gain  Gain=dt/T
  Saturation : Saturate  UpperLimit=max  LowerLimit=min
  Sum5 : Sum  Inputs=|+-
  Sum6 : Sum  Inputs=|++
  Sum7 : Sum  Inputs=+-|
  OUT : Outport
  wires:
  Constant1/1 -> Add/1
  IN/1 -> Gain2/1
  Add/1 -> Delay2/1, Saturation/1
  Sum6/1 -> Delay1/1, Add/3
  Saturation/1 -> OUT/1, Delay3/1
  Gain2/1 -> Sum5/1, Add/2
  Gain5/1 -> Sum6/1
  Delay3/1 -> Sum7/2
  Sum5/1 -> Gain5/1
  Delay1/1 -> Sum6/2
  Sum7/1 -> Sum5/2
  Delay2/1 -> Sum7/1

== system Storage_Cell/Повышающий1/PI-reg discrete I1 ==
  IN : Inport
  Add : Sum  Inputs=+++
  Constant1 : Constant  Value=First_condition
  Delay1 : Delay  DelayLength=1  InitialCondition=0  SampleTime=dt
  Delay2 : Delay  DelayLength=1  InitialCondition=0  SampleTime=dt
  Delay3 : Delay  DelayLength=1  InitialCondition=0  SampleTime=dt
  Gain2 : Gain  Gain=K
  Gain5 : Gain  Gain=dt/T
  Saturation : Saturate  UpperLimit=max  LowerLimit=min
  Sum5 : Sum  Inputs=|+-
  Sum6 : Sum  Inputs=|++
  Sum7 : Sum  Inputs=+-|
  OUT : Outport
  wires:
  Delay2/1 -> Sum7/1
  Sum7/1 -> Sum5/2
  Delay1/1 -> Sum6/2
  Sum5/1 -> Gain5/1
  Delay3/1 -> Sum7/2
  Gain5/1 -> Sum6/1
  Gain2/1 -> Add/2, Sum5/1
  Saturation/1 -> Delay3/1, OUT/1
  Sum6/1 -> Add/3, Delay1/1
  Add/1 -> Saturation/1, Delay2/1
  IN/1 -> Gain2/1
  Constant1/1 -> Add/1

== system Storage_Cell/Повышающий1/PI-reg discrete U ==
  IN : Inport
  Add : Sum  Inputs=+++
  Constant1 : Constant  Value=First_condition
  Delay1 : Delay  DelayLength=1  InitialCondition=0  SampleTime=dt
  Delay2 : Delay  DelayLength=1  InitialCondition=0  SampleTime=dt
  Delay3 : Delay  DelayLength=1  InitialCondition=0  SampleTime=dt
  Gain2 : Gain  Gain=K
  Gain5 : Gain  Gain=dt/T
  Saturation : Saturate  UpperLimit=max  LowerLimit=min
  Sum5 : Sum  Inputs=|+-
  Sum6 : Sum  Inputs=|++
  Sum7 : Sum  Inputs=+-|
  OUT : Outport
  wires:
  Delay2/1 -> Sum7/1
  Sum7/1 -> Sum5/2
  Delay1/1 -> Sum6/2
  Sum5/1 -> Gain5/1
  Delay3/1 -> Sum7/2
  Gain5/1 -> Sum6/1
  Gain2/1 -> Add/2, Sum5/1
  Saturation/1 -> Delay3/1, OUT/1
  Sum6/1 -> Add/3, Delay1/1
  Add/1 -> Saturation/1, Delay2/1
  IN/1 -> Gain2/1
  Constant1/1 -> Add/1

== system Storage_Cell/Повышающий1/PI-reg discrete U1 ==
  IN : Inport
  Add : Sum  Inputs=+++
  Constant1 : Constant  Value=First_condition
  Delay1 : Delay  DelayLength=1  InitialCondition=0  SampleTime=dt
  Delay2 : Delay  DelayLength=1  InitialCondition=0  SampleTime=dt
  Delay3 : Delay  DelayLength=1  InitialCondition=0  SampleTime=dt
  Gain2 : Gain  Gain=K
  Gain5 : Gain  Gain=dt/T
  Saturation : Saturate  UpperLimit=max  LowerLimit=min
  Sum5 : Sum  Inputs=|+-
  Sum6 : Sum  Inputs=|++
  Sum7 : Sum  Inputs=+-|
  OUT : Outport
  wires:
  Constant1/1 -> Add/1
  IN/1 -> Gain2/1
  Add/1 -> Delay2/1, Saturation/1
  Sum6/1 -> Delay1/1, Add/3
  Saturation/1 -> OUT/1, Delay3/1
  Gain2/1 -> Sum5/1, Add/2
  Gain5/1 -> Sum6/1
  Delay3/1 -> Sum7/2
  Sum5/1 -> Gain5/1
  Delay1/1 -> Sum6/2
  Sum7/1 -> Sum5/2
  Delay2/1 -> Sum7/1

== system Storage_Cell/Понижающий1/PI-reg discrete I ==
  IN : Inport
  Add : Sum  Inputs=+++
  Constant1 : Constant  Value=First_condition
  Delay1 : Delay  DelayLength=1  InitialCondition=0  SampleTime=dt
  Delay2 : Delay  DelayLength=1  InitialCondition=0  SampleTime=dt
  Delay3 : Delay  DelayLength=1  InitialCondition=0  SampleTime=dt
  Gain2 : Gain  Gain=K
  Gain5 : Gain  Gain=dt/T
  Saturation : Saturate  UpperLimit=max  LowerLimit=min
  Sum5 : Sum  Inputs=|+-
  Sum6 : Sum  Inputs=|++
  Sum7 : Sum  Inputs=+-|
  OUT : Outport
  wires:
  Delay2/1 -> Sum7/1
  Sum7/1 -> Sum5/2
  Delay1/1 -> Sum6/2
  Sum5/1 -> Gain5/1
  Delay3/1 -> Sum7/2
  Gain5/1 -> Sum6/1
  Gain2/1 -> Add/2, Sum5/1
  Saturation/1 -> Delay3/1, OUT/1
  Sum6/1 -> Add/3, Delay1/1
  Add/1 -> Saturation/1, Delay2/1
  IN/1 -> Gain2/1
  Constant1/1 -> Add/1

== system Storage_Cell/Понижающий1/PI-reg discrete U ==
  IN : Inport
  Add : Sum  Inputs=+++
  Constant1 : Constant  Value=First_condition
  Delay1 : Delay  DelayLength=1  InitialCondition=0  SampleTime=dt
  Delay2 : Delay  DelayLength=1  InitialCondition=0  SampleTime=dt
  Delay3 : Delay  DelayLength=1  InitialCondition=0  SampleTime=dt
  Gain2 : Gain  Gain=K
  Gain5 : Gain  Gain=dt/T
  Saturation : Saturate  UpperLimit=max  LowerLimit=min
  Sum5 : Sum  Inputs=|+-
  Sum6 : Sum  Inputs=|++
  Sum7 : Sum  Inputs=+-|
  OUT : Outport
  wires:
  Constant1/1 -> Add/1
  IN/1 -> Gain2/1
  Add/1 -> Delay2/1, Saturation/1
  Sum6/1 -> Delay1/1, Add/3
  Saturation/1 -> OUT/1, Delay3/1
  Gain2/1 -> Sum5/1, Add/2
  Gain5/1 -> Sum6/1
  Delay3/1 -> Sum7/2
  Sum5/1 -> Gain5/1
  Delay1/1 -> Sum6/2
  Sum7/1 -> Sum5/2
  Delay2/1 -> Sum7/1
